simulink model "Linearised_Plant_Model"  (R2020b)
settings: Solver=VariableStepAuto  StartTime=0.0  StopTime=10.0  RelTol=1e-3
settings Model: Creator=Josh_  LastModifiedBy=maria
settings DataIOCC: ReturnWorkspaceOutputs=off

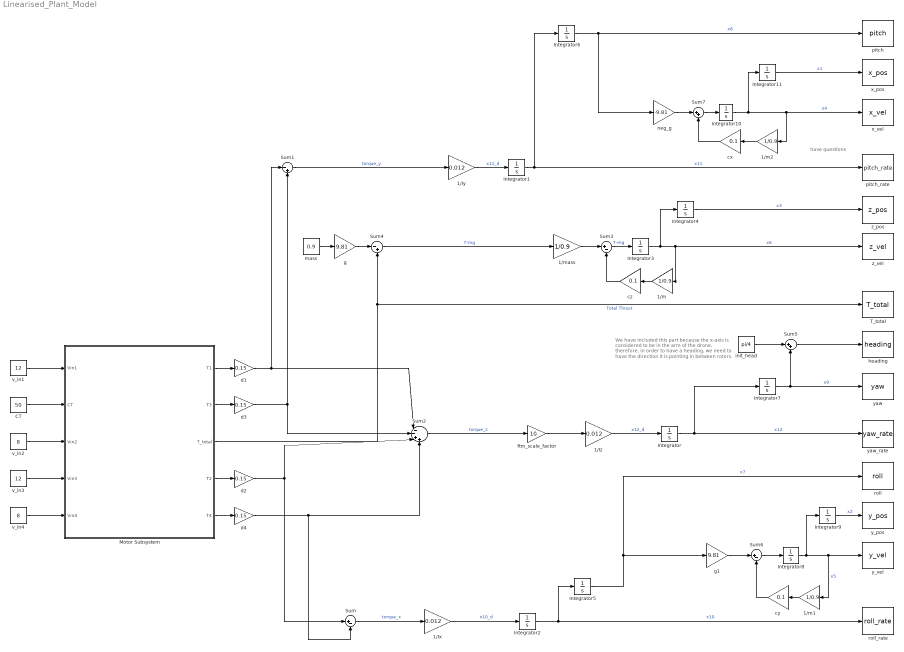
== system Linearised_Plant_Model ==
  note: We have included this part because the x-axis is considered to be in the arm of the drone, therefore, in order to have a heading, we need to have the direction it is pointing in between rotors.
  note: have questions
  1/Ix : Gain  Gain=0.012
  1/Iy : Gain  Gain=0.012
  1/Iz : Gain  Gain=0.012
  1/m : Gain  Gain=1/0.9
  1/m1 : Gain  Gain=1/0.9
  1/m2 : Gain  Gain=1/0.9
  1/mass : Gain  Gain=1/0.9
  CT : Constant  Value=50
  Integrator{,1..11} (12 alike) : Integrator
  Motor Subsystem : Subsystem
  Sum : Sum  Inputs=|+-
  Sum1 : Sum  Inputs=|-+
  Sum2 : Sum  Inputs=|--++
  Sum3 : Sum  Inputs=|+-
  Sum4 : Sum  Inputs=|-+
  Sum5 : Sum  Inputs=|++
  Sum6 : Sum  Inputs=|+-
  Sum7 : Sum  Inputs=|++
  T_total : ToWorkspace  VariableName=T_total  SaveFormat=Timeseries  SampleTime=-1
  cx : Gain  Gain=0.1
  cy : Gain  Gain=0.1
  cz : Gain  Gain=0.1
  d{1..4} (4 alike) : Gain  Gain=0.15
  ftm_scale_factor : Gain  Gain=10
  g : Gain  Gain=9.81
  g1 : Gain  Gain=9.81
  heading : ToWorkspace  VariableName=heading  SaveFormat=Timeseries  SampleTime=-1
  init_head : Constant  Value=pi/4
  mass : Constant  Value=0.9
  neg_g : Gain  Gain=-9.81
  pitch : ToWorkspace  VariableName=pitch  SaveFormat=Timeseries  SampleTime=-1
  pitch_rate : ToWorkspace  VariableName=pitch_rate  SaveFormat=Timeseries  SampleTime=-1
  roll : ToWorkspace  VariableName=roll  SaveFormat=Timeseries  SampleTime=-1
  roll_rate : ToWorkspace  VariableName=roll_rate  SaveFormat=Timeseries  SampleTime=-1
  v_in1 : Constant  Value=12
  v_in2 : Constant  Value=8
  v_in3 : Constant  Value=12
  v_in4 : Constant  Value=8
  x_pos : ToWorkspace  VariableName=x_pos  SaveFormat=Timeseries  SampleTime=-1
  x_vel : ToWorkspace  VariableName=x_vel  SaveFormat=Timeseries  SampleTime=-1
  y_pos : ToWorkspace  VariableName=y_pos  SaveFormat=Timeseries  SampleTime=-1
  y_vel : ToWorkspace  VariableName=y_vel  SaveFormat=Timeseries  SampleTime=-1
  yaw : ToWorkspace  VariableName=yaw  SaveFormat=Timeseries  SampleTime=-1
  yaw_rate : ToWorkspace  VariableName=yaw_rate  SaveFormat=Timeseries  SampleTime=-1
  z_pos : ToWorkspace  VariableName=z_pos  SaveFormat=Timeseries  SampleTime=-1
  z_vel : ToWorkspace  VariableName=z_vel  SaveFormat=Timeseries  SampleTime=-1
  wires:
  d2/1 -> Sum/1, Sum2/3
  Sum/1 -> 1/Ix/1  "torque_x"
  d1/1 -> Sum1/1, Sum2/1
  d4/1 -> Sum/2, Sum2/4
  d3/1 -> Sum2/2, Sum1/2
  Sum1/1 -> 1/Iy/1  "torque_y"
  Sum2/1 -> ftm_scale_factor/1  "torque_z"
  ftm_scale_factor/1 -> 1/Iz/1
  1/Ix/1 -> Integrator2/1  "x10_d"
  1/Iz/1 -> Integrator/1  "x12_d"
  1/Iy/1 -> Integrator1/1  "x11_d"
  Integrator/1 -> Integrator7/1, yaw_rate/1  "x12"
  Integrator1/1 -> pitch_rate/1, Integrator6/1  "x11"
  Integrator2/1 -> roll_rate/1, Integrator5/1  "x10"
  mass/1 -> g/1
  g/1 -> Sum4/1
  Integrator3/1 -> Integrator4/1, 1/m/1, z_vel/1  "x6"
  Integrator4/1 -> z_pos/1  "x3"
  Sum4/1 -> 1/mass/1  "T-mg"
  Integrator5/1 -> g1/1, roll/1  "x7"
  Integrator6/1 -> neg_g/1, pitch/1  "x8"
  Integrator7/1 -> Sum5/2, yaw/1  "x9"
  Integrator9/1 -> y_pos/1  "x2"
  Integrator10/1 -> 1/m2/1, x_vel/1, Integrator11/1  "x4"
  Integrator11/1 -> x_pos/1  "x1"
  init_head/1 -> Sum5/1
  Sum5/1 -> heading/1
  Motor Subsystem/2(T3) -> d3/1
  Motor Subsystem/5(T4) -> d4/1
  Motor Subsystem/4(T2) -> d2/1
  Motor Subsystem/1(T1) -> d1/1
  v_in1/1 -> Motor Subsystem/1(Vin1)
  CT/1 -> Motor Subsystem/2(CT)
  v_in2/1 -> Motor Subsystem/3(Vin2)
  Motor Subsystem/3(T_total) -> Sum4/2, T_total/1  "Total Thrust"
  1/mass/1 -> Sum3/1
  Sum3/1 -> Integrator3/1  "T-mg"
  1/m/1 -> cz/1
  cz/1 -> Sum3/2
  cy/1 -> Sum6/2
  1/m1/1 -> cy/1
  Integrator8/1 -> 1/m1/1, y_vel/1, Integrator9/1  "x5"
  g1/1 -> Sum6/1
  Sum6/1 -> Integrator8/1
  neg_g/1 -> Sum7/1
  Sum7/1 -> Integrator10/1
  cx/1 -> Sum7/2
  1/m2/1 -> cx/1
  v_in3/1 -> Motor Subsystem/4(Vin3)
  v_in4/1 -> Motor Subsystem/5(Vin4)

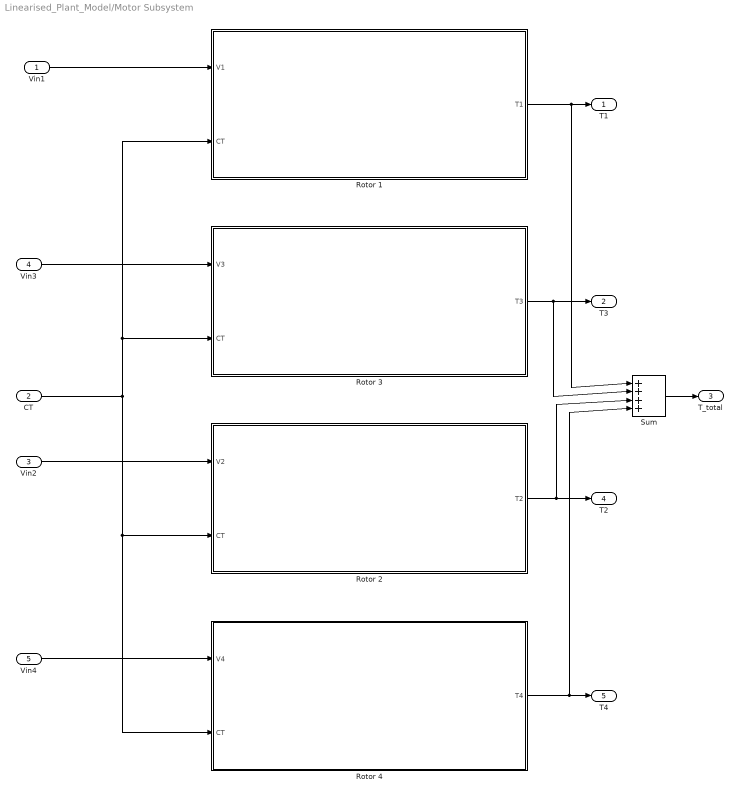
== system Linearised_Plant_Model/Motor Subsystem ==
  Vin1 : Inport
  CT : Inport  Port=2
  Vin2 : Inport  Port=3
  Vin3 : Inport  Port=4
  Vin4 : Inport  Port=5
  Rotor 1 : Subsystem
  Rotor 2 : Subsystem
  Rotor 3 : Subsystem
  Rotor 4 : Subsystem
  Sum : Sum  Inputs=|++++
  T1 : Outport
  T3 : Outport  Port=2
  T_total : Outport  Port=3
  T2 : Outport  Port=4
  T4 : Outport  Port=5
  wires:
  CT/1 -> Rotor 4/2(CT), Rotor 2/2(CT), Rotor 1/2(CT), Rotor 3/2(CT)
  Rotor 2/1(T2) -> Sum/3, T2/1
  Vin2/1 -> Rotor 2/1(V2)
  Vin1/1 -> Rotor 1/1(V1)
  Rotor 1/1(T1) -> Sum/1, T1/1
  Rotor 3/1(T3) -> Sum/2, T3/1
  Rotor 4/1(T4) -> Sum/4, T4/1
  Sum/1 -> T_total/1
  Vin3/1 -> Rotor 3/1(V3)
  Vin4/1 -> Rotor 4/1(V4)

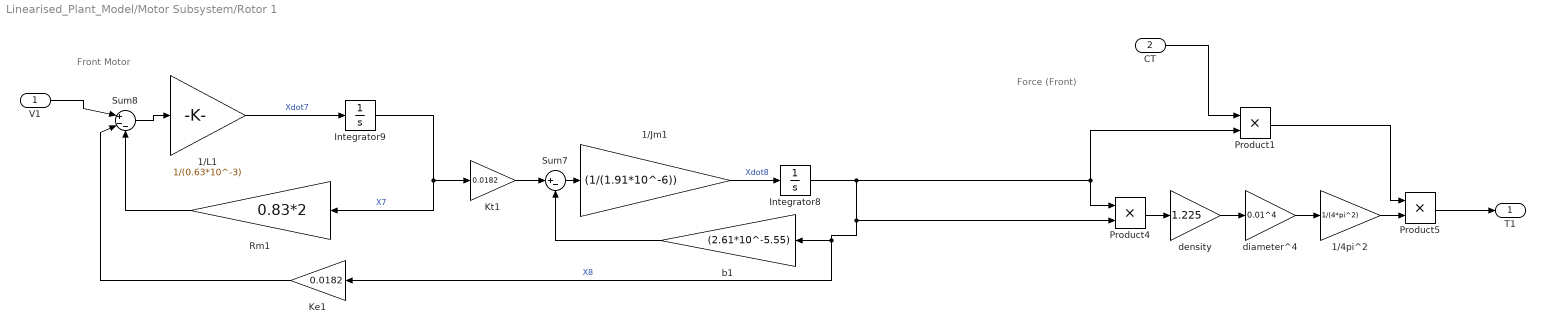
== system Linearised_Plant_Model/Motor Subsystem/Rotor 1 ==
  note: Front Motor
  note: Force (Front)
  V1 : Inport
  CT : Inport  Port=2
  1/4pi^2 : Gain  Gain=1/(4*pi^2)
  1/Jm1 : Gain  Gain=(1/(1.91*10^-6))
  1/L1 : Gain  Gain=1/(0.63*10^-3)
  Integrator8 : Integrator
  Integrator9 : Integrator
  Ke1 : Gain  Gain=0.0182
  Kt1 : Gain  Gain=0.0182
  Product1 : Product
  Product4 : Product
  Product5 : Product
  Rm1 : Gain  Gain=0.83*2
  Sum7 : Sum  Inputs=|+-
  Sum8 : Sum  Inputs=|+--
  b1 : Gain  Gain=(2.61*10^-5.55)
  density : Gain  Gain=1.225
  diameter^4 : Gain  Gain=0.01^4
  T1 : Outport
  wires:
  Rm1/1 -> Sum8/3
  1/L1/1 -> Integrator9/1  "Xdot7"
  Sum7/1 -> 1/Jm1/1
  density/1 -> diameter^4/1
  Integrator8/1 -> Ke1/1, b1/1, Product4/2, Product1/2, Product4/1  "X8"
  diameter^4/1 -> 1/4pi^2/1
  Ke1/1 -> Sum8/2
  Product4/1 -> density/1
  Integrator9/1 -> Kt1/1, Rm1/1  "X7"
  1/4pi^2/1 -> Product5/2
  Product5/1 -> T1/1
  V1/1 -> Sum8/1
  Sum8/1 -> 1/L1/1
  Kt1/1 -> Sum7/1
  1/Jm1/1 -> Integrator8/1  "Xdot8"
  Product1/1 -> Product5/1
  b1/1 -> Sum7/2
  CT/1 -> Product1/1

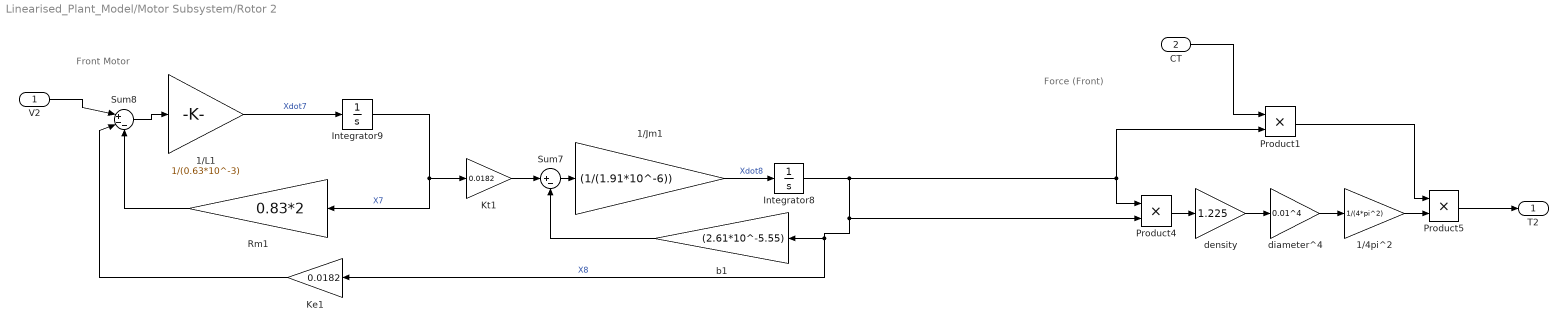
== system Linearised_Plant_Model/Motor Subsystem/Rotor 2 ==
  note: Front Motor
  note: Force (Front)
  V2 : Inport
  CT : Inport  Port=2
  1/4pi^2 : Gain  Gain=1/(4*pi^2)
  1/Jm1 : Gain  Gain=(1/(1.91*10^-6))
  1/L1 : Gain  Gain=1/(0.63*10^-3)
  Integrator8 : Integrator
  Integrator9 : Integrator
  Ke1 : Gain  Gain=0.0182
  Kt1 : Gain  Gain=0.0182
  Product1 : Product
  Product4 : Product
  Product5 : Product
  Rm1 : Gain  Gain=0.83*2
  Sum7 : Sum  Inputs=|+-
  Sum8 : Sum  Inputs=|+--
  b1 : Gain  Gain=(2.61*10^-5.55)
  density : Gain  Gain=1.225
  diameter^4 : Gain  Gain=0.01^4
  T2 : Outport
  wires:
  Rm1/1 -> Sum8/3
  1/L1/1 -> Integrator9/1  "Xdot7"
  Sum7/1 -> 1/Jm1/1
  Ke1/1 -> Sum8/2
  Integrator9/1 -> Kt1/1, Rm1/1  "X7"
  V2/1 -> Sum8/1
  Sum8/1 -> 1/L1/1
  Kt1/1 -> Sum7/1
  1/Jm1/1 -> Integrator8/1  "Xdot8"
  b1/1 -> Sum7/2
  CT/1 -> Product1/1
  Product1/1 -> Product5/1
  Product4/1 -> density/1
  1/4pi^2/1 -> Product5/2
  Integrator8/1 -> Product1/2, Product4/1, Product4/2, Ke1/1, b1/1  "X8"
  diameter^4/1 -> 1/4pi^2/1
  Product5/1 -> T2/1
  density/1 -> diameter^4/1

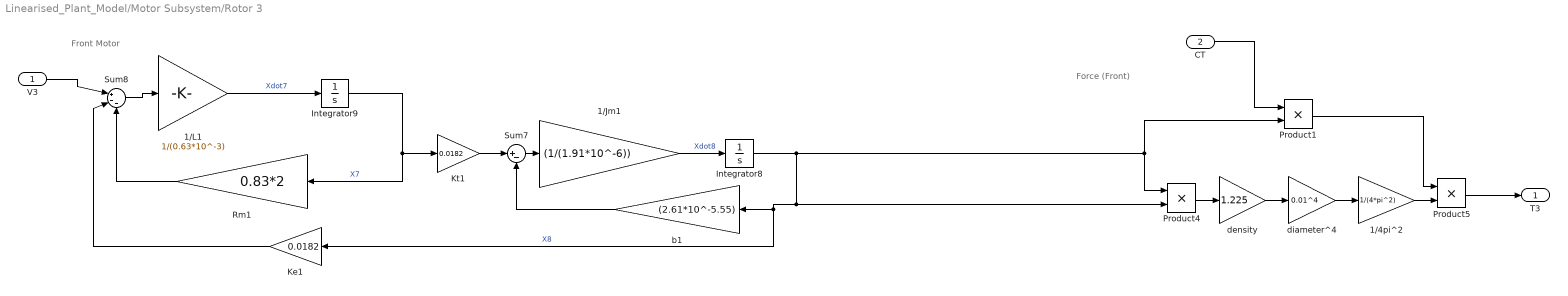
== system Linearised_Plant_Model/Motor Subsystem/Rotor 3 ==
  note: Front Motor
  note: Force (Front)
  V3 : Inport
  CT : Inport  Port=2
  1/4pi^2 : Gain  Gain=1/(4*pi^2)
  1/Jm1 : Gain  Gain=(1/(1.91*10^-6))
  1/L1 : Gain  Gain=1/(0.63*10^-3)
  Integrator8 : Integrator
  Integrator9 : Integrator
  Ke1 : Gain  Gain=0.0182
  Kt1 : Gain  Gain=0.0182
  Product1 : Product
  Product4 : Product
  Product5 : Product
  Rm1 : Gain  Gain=0.83*2
  Sum7 : Sum  Inputs=|+-
  Sum8 : Sum  Inputs=|+--
  b1 : Gain  Gain=(2.61*10^-5.55)
  density : Gain  Gain=1.225
  diameter^4 : Gain  Gain=0.01^4
  T3 : Outport
  wires:
  Rm1/1 -> Sum8/3
  1/L1/1 -> Integrator9/1  "Xdot7"
  Sum7/1 -> 1/Jm1/1
  Ke1/1 -> Sum8/2
  Integrator9/1 -> Kt1/1, Rm1/1  "X7"
  V3/1 -> Sum8/1
  Sum8/1 -> 1/L1/1
  Kt1/1 -> Sum7/1
  1/Jm1/1 -> Integrator8/1  "Xdot8"
  b1/1 -> Sum7/2
  CT/1 -> Product1/1
  Product1/1 -> Product5/1
  Product4/1 -> density/1
  1/4pi^2/1 -> Product5/2
  Integrator8/1 -> Ke1/1, b1/1, Product4/2, Product4/1, Product1/2  "X8"
  diameter^4/1 -> 1/4pi^2/1
  Product5/1 -> T3/1
  density/1 -> diameter^4/1

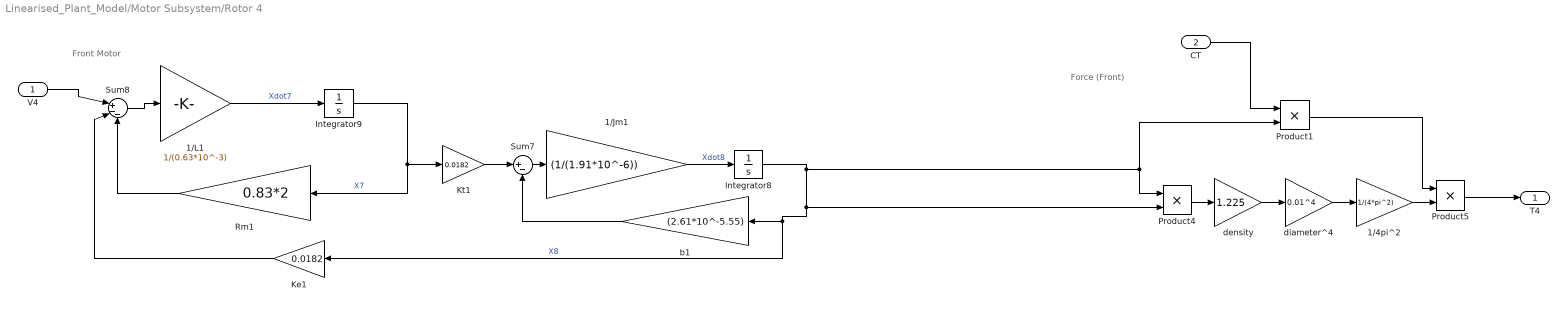
== system Linearised_Plant_Model/Motor Subsystem/Rotor 4 ==
  note: Front Motor
  note: Force (Front)
  V4 : Inport
  CT : Inport  Port=2
  1/4pi^2 : Gain  Gain=1/(4*pi^2)
  1/Jm1 : Gain  Gain=(1/(1.91*10^-6))
  1/L1 : Gain  Gain=1/(0.63*10^-3)
  Integrator8 : Integrator
  Integrator9 : Integrator
  Ke1 : Gain  Gain=0.0182
  Kt1 : Gain  Gain=0.0182
  Product1 : Product
  Product4 : Product
  Product5 : Product
  Rm1 : Gain  Gain=0.83*2
  Sum7 : Sum  Inputs=|+-
  Sum8 : Sum  Inputs=|+--
  b1 : Gain  Gain=(2.61*10^-5.55)
  density : Gain  Gain=1.225
  diameter^4 : Gain  Gain=0.01^4
  T4 : Outport
  wires:
  Rm1/1 -> Sum8/3
  1/L1/1 -> Integrator9/1  "Xdot7"
  Sum7/1 -> 1/Jm1/1
  Ke1/1 -> Sum8/2
  Integrator9/1 -> Kt1/1, Rm1/1  "X7"
  V4/1 -> Sum8/1
  Sum8/1 -> 1/L1/1
  Kt1/1 -> Sum7/1
  1/Jm1/1 -> Integrator8/1  "Xdot8"
  b1/1 -> Sum7/2
  CT/1 -> Product1/1
  Product1/1 -> Product5/1
  Product4/1 -> density/1
  1/4pi^2/1 -> Product5/2
  Integrator8/1 -> Product1/2, Product4/1, Product4/2, Ke1/1, b1/1  "X8"
  diameter^4/1 -> 1/4pi^2/1
  Product5/1 -> T4/1
  density/1 -> diameter^4/1
